simulink model "blk_tuning"  (R2017a)
settings: Solver=VariableStepAuto  StartTime=0.0  StopTime=40  MaxStep=1e-3  RelTol=1e-3
settings Model: Creator=erich  LastModifiedBy=erich

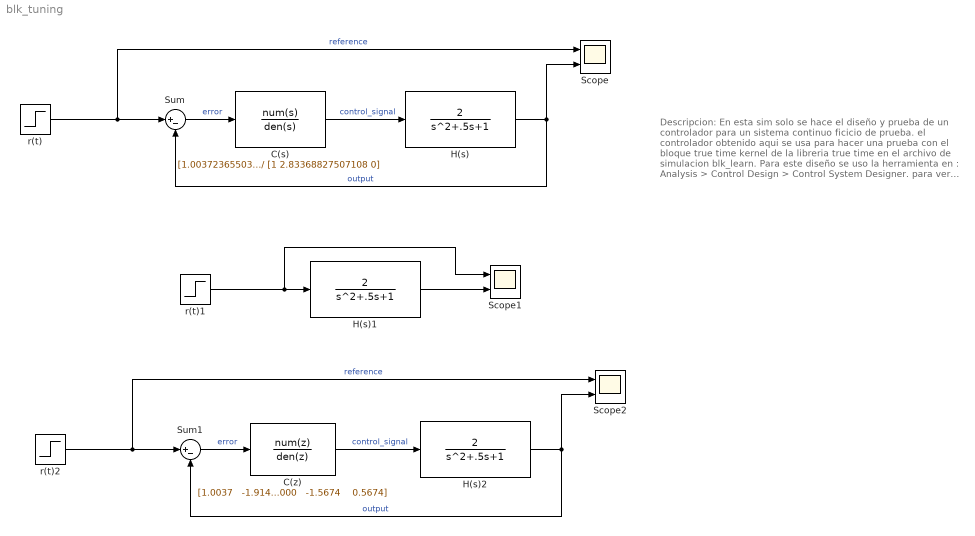
== system blk_tuning ==
  note: Descripcion:
      | En esta sim solo se hace el diseño y
      | prueba de un controlador para un
      | sistema continuo ficicio de prueba.
      | el controlador obtenido aqui se
      | usa para hacer una prueba con el
      | bloque true time kernel de la libreria
      | true time en el archivo de simulacion
      | blk_learn.
      |
      | Para este diseño se uso la herramienta
      | en :
      | Analysis > Control Design >
      | Control System Designer.
      |
      | para ver mas detalles del diseño cargar
      | la sesion em la carpeta de esta simulacion.
  C(s) : TransferFcn  Numerator=[1.00372365503441 0.501861827517207 1.00372365503441]  Denominator=[1 2.83368827507108 0]
  C(z) : DiscreteTransferFcn  Numerator="[1.0037   -1.9141    0.9410]"  Denominator="[1.0000   -1.5674    0.5674]"  SampleTime=.2
  H(s) : TransferFcn  Numerator=[2]  Denominator=[1 .5 1]
  H(s)1 : TransferFcn  Numerator=[2]  Denominator=[1 .5 1]
  H(s)2 : TransferFcn  Numerator=[2]  Denominator=[1 .5 1]
  Scope : Scope  NumInputPorts=2
  Scope1 : Scope  NumInputPorts=2
  Scope2 : Scope  NumInputPorts=2
  Sum : Sum  Inputs=|+-
  Sum1 : Sum  Inputs=|+-
  r(t) : Step  SampleTime=0
  r(t)1 : Step  SampleTime=0
  r(t)2 : Step  SampleTime=0
  wires:
  r(t)/1 -> Scope/1, Sum/1  "reference"
  H(s)/1 -> Scope/2, Sum/2  "output"
  Sum/1 -> C(s)/1  "error"
  C(s)/1 -> H(s)/1  "control_signal"
  H(s)1/1 -> Scope1/2
  r(t)1/1 -> Scope1/1, H(s)1/1
  C(z)/1 -> H(s)2/1  "control_signal"
  Sum1/1 -> C(z)/1  "error"
  H(s)2/1 -> Sum1/2, Scope2/2  "output"
  r(t)2/1 -> Sum1/1, Scope2/1  "reference"
